simulink model "Celsius_to_fahreinheit_testing"  (R2020b)
settings: Solver=VariableStepAuto  StartTime=0.0  StopTime=300.0  RelTol=1e-3
libraries: simulink x1
settings Model: Creator=Training  LastModifiedBy=Training

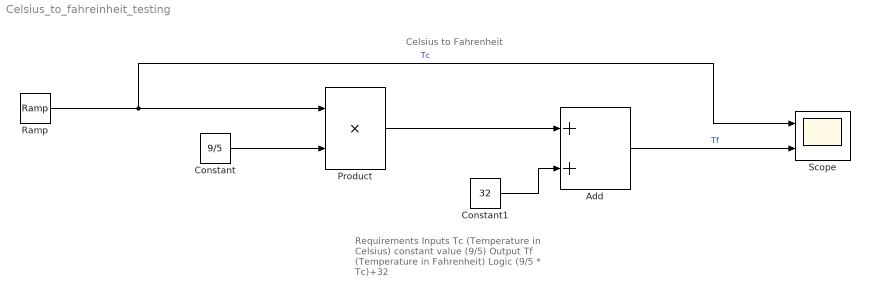
== system Celsius_to_fahreinheit_testing ==
  note: Requirements
      | Inputs
      | Tc (Temperature in Celsius)
      | constant value (9/5)
      | Output
      | Tf (Temperature in Fahrenheit)
      | Logic
      | (9/5 * Tc)+32
  note: Celsius to Fahrenheit
  Add : Sum
  Constant : Constant  Value=9/5
  Constant1 : Constant  Value=32
  Product : Product
  Ramp : simulink/Sources/Ramp  slope=1  start=0  InitialOutput=-50
  Scope : Scope  NumInputPorts=2
  wires:
  Ramp/1 -> Scope/1, Product/1  "Tc"
  Constant/1 -> Product/2
  Product/1 -> Add/1
  Constant1/1 -> Add/2
  Add/1 -> Scope/2  "Tf"
